simulink model "digital12"  (R2024a)
settings: Solver=VariableStepAuto  StartTime=0.0  StopTime=10.0  RelTol=1e-3
settings Model: Creator=tusha  LastModifiedBy=tusha

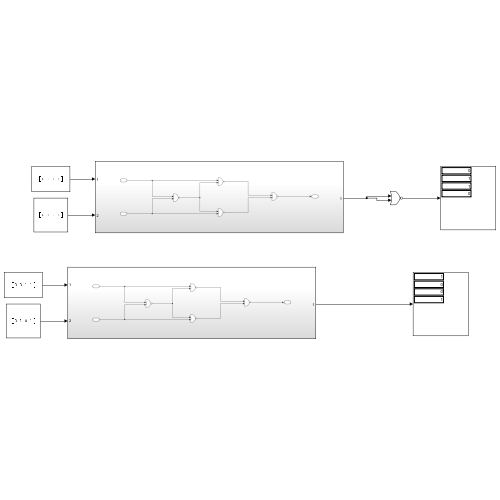
[thumbnail: Simulink's stored preview of the top-level diagram]
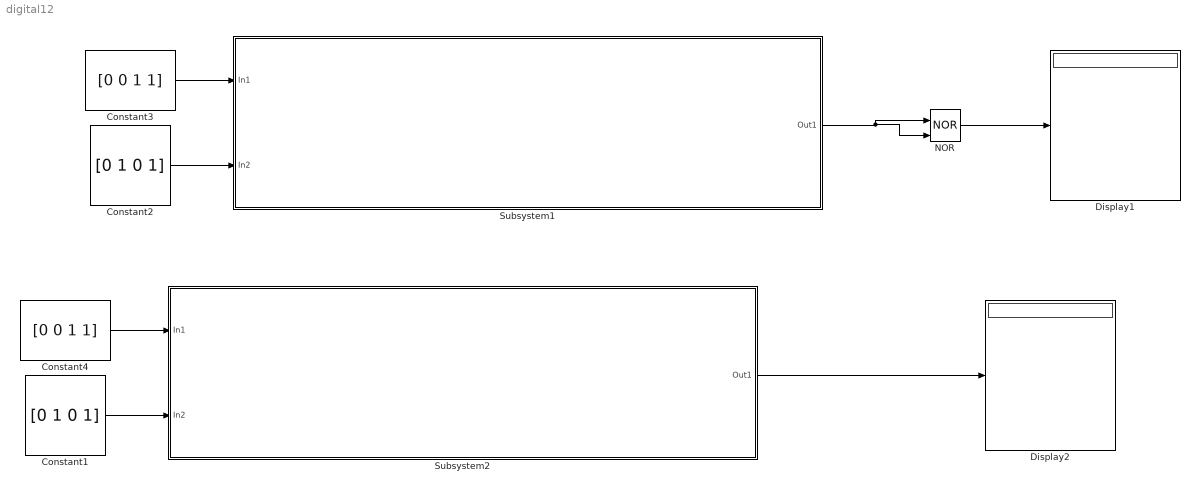
== system digital12 ==
  Constant1 : Constant  Value=[0 1 0 1]
  Constant2 : Constant  Value=[0 1 0 1]
  Constant3 : Constant  Value=[0 0 1 1]
  Constant4 : Constant  Value=[0 0 1 1]
  Display1 : Display
  Display2 : Display
  NOR : Logic  Operator=NOR  IconShape=distinctive  AllPortsSameDT=off  OutDataTypeStr=boolean
  Subsystem1 : Subsystem
  Subsystem2 : Subsystem
  wires:
  Constant2/1 -> Subsystem1/2(In2)
  Constant3/1 -> Subsystem1/1(In1)
  Subsystem1/1(Out1) -> NOR/2, NOR/1
  NOR/1 -> Display1/1
  Subsystem2/1(Out1) -> Display2/1
  Constant4/1 -> Subsystem2/1(In1)
  Constant1/1 -> Subsystem2/2(In2)

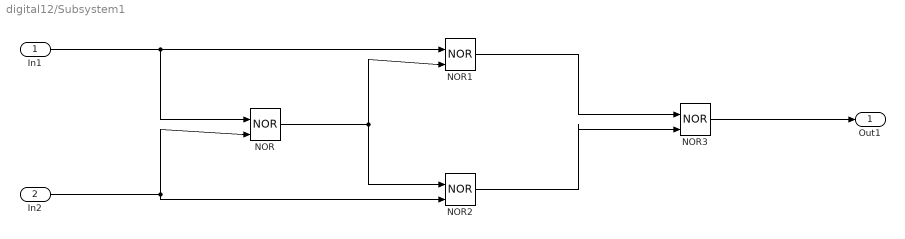
== system digital12/Subsystem1 ==
  In1 : Inport
  In2 : Inport  Port=2
  NOR{,1..3} (4 alike) : Logic  Operator=NOR  IconShape=distinctive  AllPortsSameDT=off  OutDataTypeStr=boolean
  Out1 : Outport
  wires:
  NOR/1 -> NOR2/1, NOR1/2
  NOR3/1 -> Out1/1
  In2/1 -> NOR2/2, NOR/2
  In1/1 -> NOR1/1, NOR/1
  NOR1/1 -> NOR3/1
  NOR2/1 -> NOR3/2

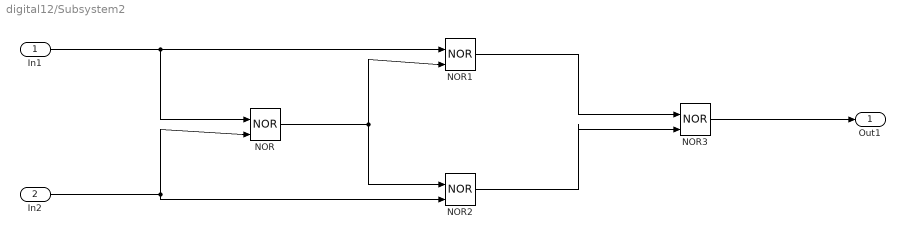
== system digital12/Subsystem2 ==
  In1 : Inport
  In2 : Inport  Port=2
  NOR{,1..3} (4 alike) : Logic  Operator=NOR  IconShape=distinctive  AllPortsSameDT=off  OutDataTypeStr=boolean
  Out1 : Outport
  wires:
  NOR/1 -> NOR2/1, NOR1/2
  NOR3/1 -> Out1/1
  In2/1 -> NOR2/2, NOR/2
  In1/1 -> NOR1/1, NOR/1
  NOR1/1 -> NOR3/1
  NOR2/1 -> NOR3/2
